simulink library "linearPathDomainPlnt_ul"  (R2018b)
settings: Solver=VariableStepAuto  StartTime=0.0  StopTime=10.0  RelTol=1e-3
settings Model: Creator=mcobb  LastModifiedBy=mcobb
settings DebuggingCC: LibraryContextMissingDiagnostic=none
settings SFSimCC: SimUseLocalCustomCode=off
settings RTWCC: RTWUseLocalCustomCode=off

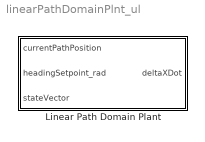
== system linearPathDomainPlnt_ul ==
  Linear Path Domain Plant : Subsystem

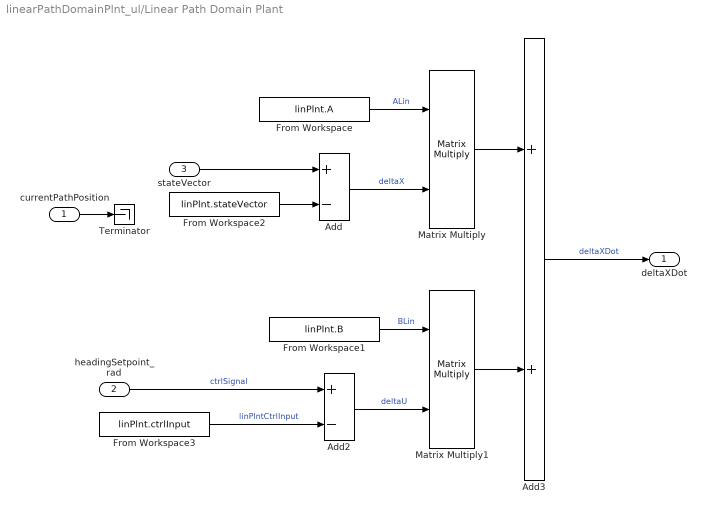
== system linearPathDomainPlnt_ul/Linear Path Domain Plant ==
  currentPathPosition : Inport  PortDimensions=1
  headingSetpoint_rad : Inport  Port=2  PortDimensions=1
  stateVector : Inport  Port=3
  Add : Sum  Inputs=+-
  Add2 : Sum  Inputs=+-
  Add3 : Sum
  From Workspace : FromWorkspace  VariableName=linPlnt.A  SampleTime=0
  From Workspace1 : FromWorkspace  VariableName=linPlnt.B  SampleTime=0
  From Workspace2 : FromWorkspace  VariableName=linPlnt.stateVector  SampleTime=0
  From Workspace3 : FromWorkspace  VariableName=linPlnt.ctrlInput  SampleTime=0
  Matrix Multiply : Product  Multiplication=Matrix(*)
  Matrix Multiply1 : Product  Multiplication=Matrix(*)
  Terminator : Terminator
  deltaXDot : Outport
  wires:
  From Workspace3/1 -> Add2/2  "linPlntCtrlInput"
  headingSetpoint_rad/1 -> Add2/1  "ctrlSignal"
  currentPathPosition/1 -> Terminator/1
  Add3/1 -> deltaXDot/1  "deltaXDot"
  From Workspace/1 -> Matrix Multiply/1  "ALin"
  Add/1 -> Matrix Multiply/2  "deltaX"
  From Workspace1/1 -> Matrix Multiply1/1  "BLin"
  Matrix Multiply1/1 -> Add3/2
  Matrix Multiply/1 -> Add3/1
  From Workspace2/1 -> Add/2
  Add2/1 -> Matrix Multiply1/2  "deltaU"
  stateVector/1 -> Add/1
